simulink model "prelab"  (R2023a)
settings: Solver=ode45  StartTime=0.0  StopTime=3  RelTol=1e-3
settings Model: Creator=Jiadong_Hong  LastModifiedBy=Jiadong_Hong

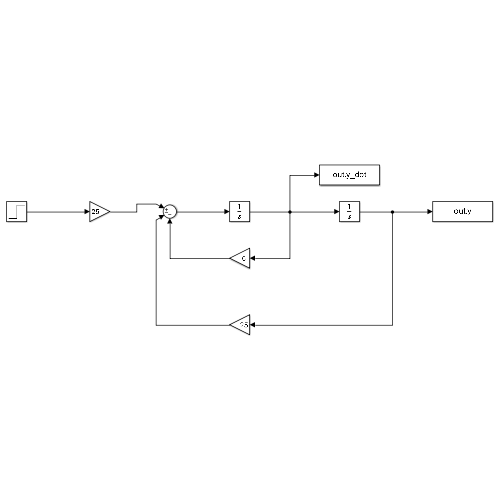
[thumbnail: Simulink's stored preview of the top-level diagram]
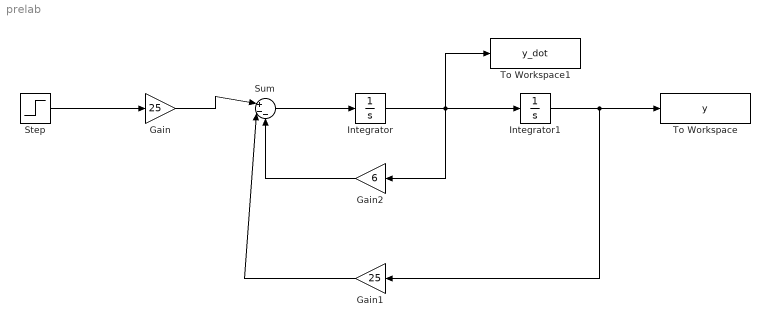
== system prelab ==
  Gain : Gain  Gain=25
  Gain1 : Gain  Gain=25
  Gain2 : Gain  Gain=6
  Integrator : Integrator
  Integrator1 : Integrator
  Step : Step  Time=0  SampleTime=0
  Sum : Sum  Inputs=|+--
  To Workspace : ToWorkspace  VariableName=y  SampleTime=-1
  To Workspace1 : ToWorkspace  VariableName=y_dot  SampleTime=-1
  wires:
  Step/1 -> Gain/1
  Gain/1 -> Sum/1
  Sum/1 -> Integrator/1
  Integrator1/1 -> Gain1/1, To Workspace/1
  Integrator/1 -> To Workspace1/1, Integrator1/1, Gain2/1
  Gain1/1 -> Sum/2
  Gain2/1 -> Sum/3
